simulink library "sm_excv_scene_lib"  (R2023a)
settings: Solver=VariableStepAuto  StartTime=0.0  StopTime=10.0  RelTol=1e-3
undefined symbols (not defined in the file): B1, B2, B3, B4, B5, B6, B7, B8, Excv, L1, L2, L3, L4, L5, L6, L7, L8, L9, Road, S1, S2, Scene, Scene_Data, SceneData, X, Y, Z
libraries: sm_lib x65, sm_tracked_vehicle_lib x47, $bdroot x45, nesl_utility x10
(part 1 of 3)
settings Model: Creator=smiller  LastModifiedBy=smiller

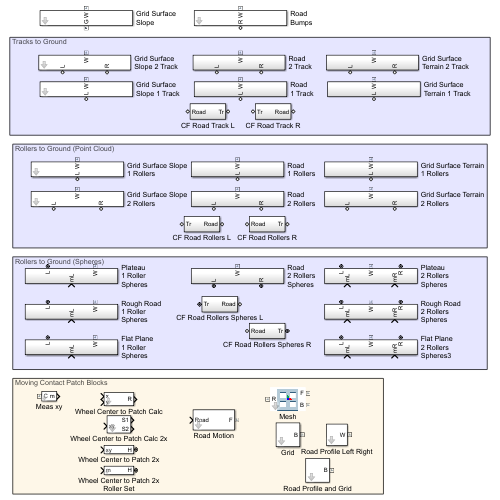
[thumbnail: Simulink's stored preview of the top-level diagram]
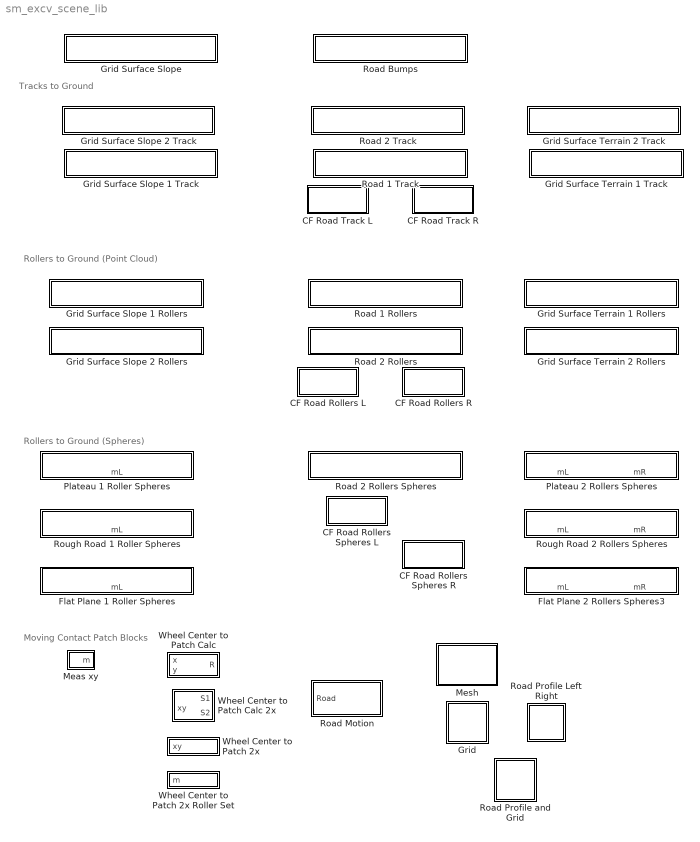
== system sm_excv_scene_lib ==
  note: Moving Contact Patch Blocks
  note: Rollers to Ground (Spheres)
  note: Tracks to Ground
  note: Rollers to Ground (Point Cloud)
  CF Road Rollers L : Subsystem
  CF Road Rollers R : Subsystem
  CF Road Rollers Spheres L : Subsystem
  CF Road Rollers Spheres R : Subsystem
  CF Road Track L : Subsystem
  CF Road Track R : Subsystem
  Flat Plane 1 Roller Spheres : Subsystem
  Flat Plane 2 Rollers Spheres3 : Subsystem
  Grid : Subsystem  VariantControl=Grid  mask(Grid){grid_x=SceneData.Grid.length, grid_y=SceneData.Grid.width, grid_z=SceneData.Grid.depth, grid_line_width=SceneData.Grid.linewidth, grid_num_sq_x=SceneData.Grid.numsquaresx, grid_num_sq_y=SceneData.Grid.numsquaresy, grid_clr=SceneData.Grid.linecolor, plane_clr=SceneData.Grid.planecolor, grid_opc=1}
      mask prompts: grid_x "Length (m) (Global x)"; grid_y "Width (m) (Global y)"; grid_z "Depth (m) (Global z)"; grid_line_width "Line width (m)"; grid_num_sq_x "Number of squares in x"; grid_num_sq_y "Number of squares in y"; grid_clr "Line Color [RGB]"; plane_clr "Plane Color [RGB]"; grid_opc "Opacity (0-1)"
      mask help: Creates a grid for use in animations.
      mask init:
      | % Derived parameters - for two perpendicular grids with num_sq-by-1 holes
      | % **Note, not num_sq_x by num_sq_y holes - better render speed with
      | % separate meshes for x and y.
      | 
      | hole_lx = (grid_x-(grid_line_width*(grid_num_sq_x+1)))/grid_num_sq_x;
      | hole_wx = (grid_y-(grid_line_width*(1+1)))/1;
      | 
      | hole_ly = (grid_y-(grid_line_width*(grid_num_sq_y+1)))/grid_num_sq_y;
      | hole_wy = (grid_x-(grid_line_width*(1+1)))/1;
  Grid Surface Slope : Subsystem  mask{road_len=Scene.Slope.road_len, road_wid=Scene.Slope.road_wid, slope_run=Scene.Slope.slope_run, slope_rise=Scene.Slope.slope_rise, slope_x0=Scene.Slope.slope_start, slope_xres=Scene.Slope.slope_xres, surface_clr=Scene.Slope.clr, surface_opc=Scene.Slope.opc}
      mask prompts: road_len "Road Length (m)"; road_wid "Road Width (m)"; slope_run "Slope Run(m)"; slope_rise "Slope Rise (m)"; slope_x0 "Slope Start (m)"; slope_xres "Slope Resolution (m)"; surface_clr "Color [R G B] (0-1)"; surface_opc "Opacity (0-1)"
      mask init:
      | gs_data = Grid_Surface_Data_Slope(road_len, road_wid, slope_run, slope_rise, slope_x0, slope_xres);
      mask TypeOptions surface_clr: Grid Surface/GraphicDiffuseColor
      mask TypeOptions surface_opc: Grid Surface/GraphicOpacity
  Grid Surface Slope 1 Track : Subsystem  mask{road_len=Scene.Slope.road_len, road_wid=Scene.Slope.road_wid, slope_rise=Scene.Slope.slope_rise, slope_run=Scene.Slope.slope_run, slope_x0=Scene.Slope.slope_start, slope_xres=Scene.Slope.slope_xres, surface_clr=Scene.Slope.clr, surface_opc=Scene.Slope.opc, K_Road=Scene.Contact.Terrain.K, B_Road=Scene.Contact.Terrain.B, TW_Road=Scene.Contact.Terrain.TW, F_dyn_Road=Scene.Contact.Terrain.mud, F_stat_Road=Scene.Contact.Terrain.mus, CV_Road=Scene.Contact.Terrain.CV}
      mask prompts: road_len "Road Length (m)"; road_wid "Road Width (m)"; slope_rise "Slope Rise (m)"; slope_run "Slope Run(m)"; slope_x0 "Slope Start (m)"; slope_xres "Slope Resolution (m)"; surface_clr "Color [R G B] (0-1)"; surface_opc "Opacity (0-1)"; K_Road "Normal Stiffness (N/m)"; B_Road "Normal Damping (N/(m/s))"; TW_Road "Normal Transition Width (m)"; F_dyn_Road "Coefficient of Dynamic Friction"; F_stat_Road "Coefficient of Static Friction"; CV_Road "Critical Velocity (m/s)"
      mask TypeOptions road_len:
      | Grid Surface
      | Slope/road_len
      mask TypeOptions road_wid:
      | Grid Surface
      | Slope/road_wid
      mask TypeOptions slope_rise:
      | Grid Surface
      | Slope/slope_rise
      mask TypeOptions slope_run:
      | Grid Surface
      | Slope/slope_run
      mask TypeOptions slope_x0:
      | Grid Surface
      | Slope/slope_x0
      mask TypeOptions slope_xres:
      | Grid Surface
      | Slope/slope_xres
      mask TypeOptions surface_clr:
      | Grid Surface
      | Slope/surface_clr
      mask TypeOptions surface_opc:
      | Grid Surface
      | Slope/surface_opc
      mask TypeOptions K_Road: CF Track Terrain L/K_Road
      mask TypeOptions B_Road: CF Track Terrain L/B_Road
      mask TypeOptions TW_Road: CF Track Terrain L/TW_Road
      mask TypeOptions F_dyn_Road: CF Track Terrain L/F_dyn_Road
      mask TypeOptions F_stat_Road: CF Track Terrain L/F_stat_Road
      mask TypeOptions CV_Road: CF Track Terrain L/CV_Road
      mask DialogControl cont_slope Prompt: Slope
      mask DialogControl cont_contact Prompt: Contact
  Grid Surface Slope 2 Track : Subsystem  mask{road_len=Scene.Slope.road_len, road_wid=Scene.Slope.road_wid, slope_rise=Scene.Slope.slope_rise, slope_run=Scene.Slope.slope_run, slope_x0=Scene.Slope.slope_start, slope_xres=Scene.Slope.slope_xres, surface_clr=Scene.Slope.clr, surface_opc=Scene.Slope.opc, TW_Road=Scene.Contact.Terrain.TW, B_Road=Scene.Contact.Terrain.B, K_Road=Scene.Contact.Terrain.K, F_dyn_Road=Scene.Contact.Terrain.mud, F_stat_Road=Scene.Contact.Terrain.mus, CV_Road=Scene.Contact.Terrain.CV}
      mask prompts: road_len "Road Length (m)"; road_wid "Road Width (m)"; slope_rise "Slope Rise (m)"; slope_run "Slope Run(m)"; slope_x0 "Slope Start (m)"; slope_xres "Slope Resolution (m)"; surface_clr "Color [R G B] (0-1)"; surface_opc "Opacity (0-1)"; TW_Road "Normal Transition Width (m)"; B_Road "Normal Damping (N/(m/s))"; K_Road "Normal Stiffness (N/m)"; F_dyn_Road "Coefficient of Dynamic Friction"; F_stat_Road "Coefficient of Static Friction"; CV_Road "Critical Velocity (m/s)"
      mask TypeOptions road_len:
      | Grid Surface
      | Slope/road_len
      mask TypeOptions road_wid:
      | Grid Surface
      | Slope/road_wid
      mask TypeOptions slope_rise:
      | Grid Surface
      | Slope/slope_rise
      mask TypeOptions slope_run:
      | Grid Surface
      | Slope/slope_run
      mask TypeOptions slope_x0:
      | Grid Surface
      | Slope/slope_x0
      mask TypeOptions slope_xres:
      | Grid Surface
      | Slope/slope_xres
      mask TypeOptions surface_clr:
      | Grid Surface
      | Slope/surface_clr
      mask TypeOptions surface_opc:
      | Grid Surface
      | Slope/surface_opc
      mask TypeOptions TW_Road: CF Track Terrain L/TW_Road | CF Track Terrain R/TW_Road
      mask TypeOptions B_Road: CF Track Terrain L/B_Road | CF Track Terrain R/B_Road
      mask TypeOptions K_Road: CF Track Terrain L/K_Road | CF Track Terrain R/K_Road
      mask TypeOptions F_dyn_Road: CF Track Terrain L/F_dyn_Road | CF Track Terrain R/F_dyn_Road
      mask TypeOptions F_stat_Road: CF Track Terrain L/F_stat_Road | CF Track Terrain R/F_stat_Road
      mask TypeOptions CV_Road: CF Track Terrain L/CV_Road | CF Track Terrain R/CV_Road
      mask DialogControl cont_slope Prompt: Slope
      mask DialogControl cont_contact Prompt: Contact
  Grid Surface Terrain 1 Track : Subsystem
  Grid Surface Terrain 2 Track : Subsystem
  Grid Surface Slope 1 Rollers : Subsystem  mask{road_len=Scene.Slope.road_len, road_wid=Scene.Slope.road_wid, slope_rise=Scene.Slope.slope_rise, slope_run=Scene.Slope.slope_run, slope_x0=Scene.Slope.slope_start, slope_xres=Scene.Slope.slope_xres, surface_clr=Scene.Slope.clr, surface_opc=Scene.Slope.opc, K_Road=Scene.Contact.Terrain.K, B_Road=Scene.Contact.Terrain.B, TW_Road=Scene.Contact.Terrain.TW, F_dyn_Road=Scene.Contact.Terrain.mud, F_stat_Road=Scene.Contact.Terrain.mus, CV_Road=Scene.Contact.Terrain.CV}
      mask prompts: road_len "Road Length (m)"; road_wid "Road Width (m)"; slope_rise "Slope Rise (m)"; slope_run "Slope Run(m)"; slope_x0 "Slope Start (m)"; slope_xres "Slope Resolution (m)"; surface_clr "Color [R G B] (0-1)"; surface_opc "Opacity (0-1)"; K_Road "Normal Stiffness (N/m)"; B_Road "Normal Damping (N/(m/s))"; TW_Road "Normal Transition Width (m)"; F_dyn_Road "Coefficient of Dynamic Friction"; F_stat_Road "Coefficient of Static Friction"; CV_Road "Critical Velocity (m/s)"
      mask TypeOptions road_len:
      | Grid Surface
      | Slope/road_len
      mask TypeOptions road_wid:
      | Grid Surface
      | Slope/road_wid
      mask TypeOptions slope_rise:
      | Grid Surface
      | Slope/slope_rise
      mask TypeOptions slope_run:
      | Grid Surface
      | Slope/slope_run
      mask TypeOptions slope_x0:
      | Grid Surface
      | Slope/slope_x0
      mask TypeOptions slope_xres:
      | Grid Surface
      | Slope/slope_xres
      mask TypeOptions surface_clr:
      | Grid Surface
      | Slope/surface_clr
      mask TypeOptions surface_opc:
      | Grid Surface
      | Slope/surface_opc
      mask TypeOptions K_Road: CF Track Terrain L/K_Road
      mask TypeOptions B_Road: CF Track Terrain L/B_Road
      mask TypeOptions TW_Road: CF Track Terrain L/TW_Road
      mask TypeOptions F_dyn_Road: CF Track Terrain L/F_dyn_Road
      mask TypeOptions F_stat_Road: CF Track Terrain L/F_stat_Road
      mask TypeOptions CV_Road: CF Track Terrain L/CV_Road
      mask DialogControl cont_slope Prompt: Slope
      mask DialogControl cont_contact Prompt: Contact
  Grid Surface Slope 2 Rollers : Subsystem  mask{road_len=Scene.Slope.road_len, road_wid=Scene.Slope.road_wid, slope_rise=Scene.Slope.slope_rise, slope_run=Scene.Slope.slope_run, slope_x0=Scene.Slope.slope_start, slope_xres=Scene.Slope.slope_xres, surface_clr=Scene.Slope.clr, surface_opc=Scene.Slope.opc, K_Road=Scene.Contact.Terrain.K, B_Road=Scene.Contact.Terrain.B, TW_Road=Scene.Contact.Terrain.TW, F_dyn_Road=Scene.Contact.Terrain.mud, F_stat_Road=Scene.Contact.Terrain.mus, CV_Road=Scene.Contact.Terrain.CV}
      mask prompts: road_len "Road Length (m)"; road_wid "Road Width (m)"; slope_rise "Slope Rise (m)"; slope_run "Slope Run(m)"; slope_x0 "Slope Start (m)"; slope_xres "Slope Resolution (m)"; surface_clr "Color [R G B] (0-1)"; surface_opc "Opacity (0-1)"; K_Road "Normal Stiffness (N/m)"; B_Road "Normal Damping (N/(m/s))"; TW_Road "Normal Transition Width (m)"; F_dyn_Road "Coefficient of Dynamic Friction"; F_stat_Road "Coefficient of Static Friction"; CV_Road "Critical Velocity (m/s)"
      mask TypeOptions road_len:
      | Grid Surface
      | Slope/road_len
      mask TypeOptions road_wid:
      | Grid Surface
      | Slope/road_wid
      mask TypeOptions slope_rise:
      | Grid Surface
      | Slope/slope_rise
      mask TypeOptions slope_run:
      | Grid Surface
      | Slope/slope_run
      mask TypeOptions slope_x0:
      | Grid Surface
      | Slope/slope_x0
      mask TypeOptions slope_xres:
      | Grid Surface
      | Slope/slope_xres
      mask TypeOptions surface_clr:
      | Grid Surface
      | Slope/surface_clr
      mask TypeOptions surface_opc:
      | Grid Surface
      | Slope/surface_opc
      mask TypeOptions K_Road: CF Track Terrain L/K_Road
      mask TypeOptions B_Road: CF Track Terrain L/B_Road
      mask TypeOptions TW_Road: CF Track Terrain L/TW_Road
      mask TypeOptions F_dyn_Road: CF Track Terrain L/F_dyn_Road
      mask TypeOptions F_stat_Road: CF Track Terrain L/F_stat_Road
      mask TypeOptions CV_Road: CF Track Terrain L/CV_Road
      mask DialogControl cont_slope Prompt: Slope
      mask DialogControl cont_contact Prompt: Contact
  Grid Surface Terrain 1 Rollers : Subsystem
  Grid Surface Terrain 2 Rollers : Subsystem
  Meas xy : Subsystem  mask(Measure Cartesian Location of two frames){whl_offset=Excv.Shoe.w}
      mask prompts: whl_offset "Frame Offset"
      mask help: Measure position of two frames. Frames are separated by a distance along their common z-axis.
  Mesh : Subsystem  mask(Rectangular Mesh){mesh_lenx=0.6, mesh_leny=0.4, mesh_hx=0.18, mesh_hy=0.18, mesh_numhx=3, mesh_numhy=2, mesh_thickness=0.02, mesh_rho=7000, mesh_color=[0 0.4 0.6], mesh_opc=1}
      mask prompts: mesh_thickness "Thickness (m)"; mesh_rho "Density (kg/m^3)"; mesh_color "Color [RGB]"; mesh_opc "Opacity (0-1)"
      mask help: Rectangular mesh. Define outer dimensions, dimensions of holes, and thickness. R port is at the CG. Thickness defines the distance of the F frame from the B frame along the z-axis.
      mask init:
      | mesh_xsec = sm_extr_data_mesh(mesh_lenx, mesh_leny, mesh_numhx, mesh_numhy, mesh_hx, mesh_hy);
      mask DialogControl Control12 Prompt: Plot Profile
      mask DialogControl Control12 Callback:
      | v = get_param(gcb,'MaskWSVariables');
      | getMaskValue = containers.Map({v.Name}',{v.Value}');
      | evalin('base',...
      |     sprintf('Extr_Data_Mesh(%s,%s,%s,%s,%s,%s,''%s'');',...
      |     num2str(getMaskValue('mesh_lenx')),...
      |     num2str(getMaskValue('mesh_leny')),...
      |     num2str(getMaskValue('mesh_numhx')),...
      |     num2str(getMaskValue('mesh_numhy')),...
      |     num2str(getMaskValue('mesh_hx')),...
      |     num2str(getMaskValue('mesh_hy')),'plot'));
      mask DialogControl Control7 Prompt: X
      mask DialogControl Control8 Prompt: Y
      mask DialogControl Control9 Prompt: Mesh Length (m)
      mask DialogControl Control11 Prompt: Hole Length (m)
      mask DialogControl Control10 Prompt: Number of Holes
      mask Display: image('sm_parts_mesh_image.png');
  Plateau 1 Roller Spheres : Subsystem
  Plateau 2 Rollers Spheres : Subsystem
  Road 1 Rollers : Subsystem
  Road 1 Track : Subsystem
  Road 2 Rollers : Subsystem
  Road 2 Rollers Spheres : Subsystem
  Road 2 Track : Subsystem
  Road Bumps : Subsystem  mask{road_x=Scene.Road.len, road_y=Scene.Road.wid, road_z=Scene.Road.hgt, bump_x=Scene.Road.Bump.len, bump_y=Scene.Road.Bump.wid, bump_z=Scene.Road.Bump.hgt, bloc_y=Scene.Road.Bump.offsety, bloc_z=Scene.Road.Bump.offsetz, bump_x0=Scene.Road.Bump.startx, bloc_dx=Scene.Road.Bump.deltax}
      mask prompts: road_x "Length (m)"; road_y "Width (m)"; road_z "Thickness (m)"; bump_x "Length (m)"; bump_y "Width (m)"; bump_z "Height (m)"; bloc_y "Offset y (m)"; bloc_z "Offset z (m)"; bump_x0 "Start x (m)"; bloc_dx "Spacing x (m)"
      mask DialogControl cont_road Prompt: Road
      mask DialogControl cont_bump_dim Prompt: Bump
      mask DialogControl cont_bump_offset Prompt: Bump Offset
  Road Motion : Subsystem  mask(Position Infinite Plane){}
      mask help: Positions and orients Infinite Plane based on input signal. Abstract method of modeling objects contacting uneven terrain.
  Road Profile Left Right : Subsystem  mask(Left and Right Paths for Wheels.){RDF_Polyline=Scene_Data.Plateau}
      mask prompts: RDF_Polyline "RDF Polyline (structure)"
      mask help: Creates left and right straightline paths for wheels as an extrusion. Look under mask to see the format of the structure required.
  Road Profile and Grid : Subsystem  VariantControl=Plateau  mask(Display Wheel Paths and Grid){RDF_Polyline=Scene.Plateau, grid_z_offset=-0.2, grid_x=Scene.Grid.length, grid_y=Scene.Grid.width, grid_z=Scene.Grid.depth, grid_line_width=Scene.Grid.linewidth, grid_num_sq_x=Scene.Grid.numsquaresx, grid_num_sq_y=Scene.Grid.numsquaresy, plane_clr=Scene.Grid.planecolor, grid_clr=Scene.Grid.linecolor, grid_opc=1}
      mask prompts: RDF_Polyline "Road Data (structure)"; grid_z_offset "Offset Grid in z (m)"; grid_x "Length (m) (Global x)"; grid_y "Width (m) (Global y)"; grid_z "Depth (m) (Global z)"; grid_line_width "Line width (m)"; grid_num_sq_x "Number of squares in x"; grid_num_sq_y "Number of squares in y"; plane_clr "Plane Color [RGB]"; grid_clr "Line Color [RGB]"; grid_opc "Opacity (0-1)"
      mask help: Display wheel paths and grid.
      mask init: same as sm_excv_scene_lib/Grid
      mask TypeOptions RDF_Polyline: Plateau/RDF_Polyline
      mask TypeOptions grid_x: Grid/grid_x
      mask TypeOptions grid_y: Grid/grid_y
      mask TypeOptions grid_z: Grid/grid_z
      mask TypeOptions grid_line_width: Grid/grid_line_width
      mask TypeOptions grid_num_sq_x: Grid/grid_num_sq_x
      mask TypeOptions grid_num_sq_y: Grid/grid_num_sq_y
      mask TypeOptions plane_clr: Grid/plane_clr
      mask TypeOptions grid_clr: Grid/grid_clr
      mask TypeOptions grid_opc: Grid/grid_opc
      mask DialogControl cont_grid Prompt: Grid Parameters
  Rough Road 1 Roller Spheres : Subsystem
  Rough Road 2 Rollers Spheres : Subsystem
  Wheel Center to Patch 2x : Subsystem  mask(Wheel Center to Patch Height and Pitch, Infinite Planes){road_pz_x=Scene.Plateau.Road.pzLUT.px, road_pz_z=Scene.Plateau.Road.pzLUT.pz(:,1), road_qy_x=Scene.Plateau.Road.qyLUT.px, road_qy_qy=Scene.Plateau.Road.qyLUT.qy(:,1), tfilter=0.01, patch_clr=[0.5 0.5 0.5], patch_opc=0.25, patch_x=1, patch_y=1, NormalStiffness=Scene.Contact.Terrain.K, NormalDamping=Scene.Contact.Terrain.B, NormalTransitionRegionWidth=Scene.Contact.Terrain.TW, CoefficientOfDynamicFriction=Scene.Contact.Terrain.mud, CoefficientOfStaticFriction=Scene.Contact.Terrain.mus, FrictionalCriticalVelocity=Scene.Contact.Terrain.CV}
      mask prompts: road_pz_x "Road Distances (m)"; road_pz_z "Road Heights (m)"; road_qy_x "Road Distances(m)"; road_qy_qy "Road Pitch (m)"; tfilter "Filter Constant (seconds)"; patch_clr "Color [R G B] (0-1)"; patch_opc "Opacity (0-1)"; patch_x "Patch Length x (m)"; patch_y "Patch Length y (m)"; NormalStiffness "Normal Stiffness (N/m)"; NormalDamping "Normal Damping (N/(m/s))"; NormalTransitionRegionWidth "Normal Transition Width (m)"; CoefficientOfDynamicFriction "Coefficient of Dynamic Friction"; CoefficientOfStaticFriction "Coefficient of Static Friction"; FrictionalCriticalVelocity "Critical Velocity (m/s)"
      mask help: Find contact patch height and pitch using a lookup table, where the inputs are the x-y location of two frames. The output is a Simscape Bus with the geometry ports for Infinite Planes positioned and pitched for the two input frame locations.
      mask TypeOptions road_pz_x:
      | Wheel Center
      | to Patch/road_pz_x
      mask TypeOptions road_pz_z:
      | Wheel Center
      | to Patch/road_pz_z
      mask TypeOptions road_qy_x:
      | Wheel Center
      | to Patch/road_qy_x
      mask TypeOptions road_qy_qy:
      | Wheel Center
      | to Patch/road_qy_qy
      mask TypeOptions tfilter:
      | Wheel Center
      | to Patch/tfilter
      mask TypeOptions patch_clr: Infinite Plane1/GraphicDiffuseColor | Infinite Plane2/GraphicDiffuseColor
      mask TypeOptions patch_opc: Infinite Plane1/GraphicOpacity | Infinite Plane2/GraphicOpacity
      mask TypeOptions patch_x: Infinite Plane1/GraphicPlaneWidth | Infinite Plane2/GraphicPlaneWidth
      mask TypeOptions patch_y: Infinite Plane1/GraphicPlaneHeight | Infinite Plane2/GraphicPlaneHeight
      mask TypeOptions NormalStiffness: CF Track Terrain1/NormalStiffness | CF Track Terrain2/NormalStiffness
      mask TypeOptions NormalDamping: CF Track Terrain1/NormalDamping | CF Track Terrain2/NormalDamping
      mask TypeOptions NormalTransitionRegionWidth: CF Track Terrain1/NormalTransitionRegionWidth | CF Track Terrain2/NormalTransitionRegionWidth
      mask TypeOptions CoefficientOfDynamicFriction: CF Track Terrain1/CoefficientOfDynamicFriction | CF Track Terrain2/CoefficientOfDynamicFriction
      mask TypeOptions CoefficientOfStaticFriction: CF Track Terrain1/CoefficientOfStaticFriction | CF Track Terrain2/CoefficientOfStaticFriction
      mask TypeOptions FrictionalCriticalVelocity: CF Track Terrain1/FrictionalCriticalVelocity | CF Track Terrain2/FrictionalCriticalVelocity
      mask DialogControl cont_surface Prompt: Surface
      mask DialogControl cont_patchvis Prompt: Patch Visual
      mask DialogControl cont_contact Prompt: Contact
  Wheel Center to Patch 2x Roller Set : Subsystem  mask(Wheel Center to Patch Height and Pitch, All Rollers){road_pz_x=Scene.Plateau.Road.pzLUT.px, road_pz_z=Scene.Plateau.Road.pzLUT.pz(:,1), road_qy_x=Scene.Plateau.Road.qyLUT.px, road_qy_qy=Scene.Plateau.Road.qyLUT.qy(:,1), tfilter=0.01, NormalStiffness=Scene.Contact.Terrain.K, NormalDamping=Scene.Contact.Terrain.B, NormalTransitionRegionWidth=Scene.Contact.Terrain.TW, CoefficientOfDynamicFriction=Scene.Contact.Terrain.mud, CoefficientOfStaticFriction=Scene.Contact.Terrain.mus, FrictionalCriticalVelocity=Scene.Contact.Terrain.CV, patch_x=1, patch_y=1, patch_clr=[0.5 0.5 0.5], patch_opc=0.25}
      mask prompts: road_pz_x "Road Distances (m)"; road_pz_z "Road Heights (m)"; road_qy_x "Road Distances(m)"; road_qy_qy "Road Pitch (m)"; tfilter "Filter Constant (seconds)"; NormalStiffness "Normal Stiffness (N/m)"; NormalDamping "Normal Damping (N/(m/s))"; NormalTransitionRegionWidth "Normal Transition Width (m)"; CoefficientOfDynamicFriction "Coefficient of Dynamic Friction"; CoefficientOfStaticFriction "Coefficient of Static Friction"; FrictionalCriticalVelocity "Critical Velocity (m/s)"; patch_x "Patch Length x (m)"; patch_y "Patch Length y (m)"; patch_clr "Color [R G B] (0-1)"; patch_opc "Opacity (0-1)"
      mask help: Find contact patch height and pitch using a lookup table, where the inputs are the x-y location of two frames. The output is a Simscape Bus with the geometry ports for Infinite Planes positioned and pitched for all input frame locations.
      mask TypeOptions road_pz_x: Wheel Center to Patch Contact 1/road_pz_x | Wheel Center to Patch Contact 2/road_pz_x | Wheel Center to Patch Contact 3/road_pz_x | Wheel Center to Patch Contact 4/road_pz_x | Wheel Center to Patch Contact 5/road_pz_x | Wheel Center to Patch Contact 6/road_pz_x | Wheel Center to Patch Contact 7/road_pz_x | Wheel Center to Patch Contact 8/road_pz_x | Wheel Center to Patch Contact 9/road_pz_x
      mask TypeOptions road_pz_z: Wheel Center to Patch Contact 1/road_pz_z | Wheel Center to Patch Contact 2/road_pz_z | Wheel Center to Patch Contact 3/road_pz_z | Wheel Center to Patch Contact 4/road_pz_z | Wheel Center to Patch Contact 5/road_pz_z | Wheel Center to Patch Contact 6/road_pz_z | Wheel Center to Patch Contact 7/road_pz_z | Wheel Center to Patch Contact 8/road_pz_z | Wheel Center to Patch Contact 9/road_pz_z
      mask TypeOptions road_qy_x: Wheel Center to Patch Contact 1/road_qy_x | Wheel Center to Patch Contact 2/road_qy_x | Wheel Center to Patch Contact 3/road_qy_x | Wheel Center to Patch Contact 4/road_qy_x | Wheel Center to Patch Contact 5/road_qy_x | Wheel Center to Patch Contact 6/road_qy_x | Wheel Center to Patch Contact 7/road_qy_x | Wheel Center to Patch Contact 8/road_qy_x | Wheel Center to Patch Contact 9/road_qy_x
      mask TypeOptions road_qy_qy: Wheel Center to Patch Contact 1/road_qy_qy | Wheel Center to Patch Contact 2/road_qy_qy | Wheel Center to Patch Contact 3/road_qy_qy | Wheel Center to Patch Contact 4/road_qy_qy | Wheel Center to Patch Contact 5/road_qy_qy | Wheel Center to Patch Contact 6/road_qy_qy | Wheel Center to Patch Contact 7/road_qy_qy | Wheel Center to Patch Contact 8/road_qy_qy | Wheel Center to Patch Contact 9/road_qy_qy
      mask TypeOptions tfilter: Wheel Center to Patch Contact 1/tfilter | Wheel Center to Patch Contact 2/tfilter | Wheel Center to Patch Contact 3/tfilter | Wheel Center to Patch Contact 4/tfilter | Wheel Center to Patch Contact 5/tfilter | Wheel Center to Patch Contact 6/tfilter | Wheel Center to Patch Contact 7/tfilter | Wheel Center to Patch Contact 8/tfilter | Wheel Center to Patch Contact 9/tfilter
      mask TypeOptions NormalStiffness: Wheel Center to Patch Contact 1/NormalStiffness | Wheel Center to Patch Contact 2/NormalStiffness | Wheel Center to Patch Contact 3/NormalStiffness | Wheel Center to Patch Contact 4/NormalStiffness | Wheel Center to Patch Contact 5/NormalStiffness | Wheel Center to Patch Contact 6/NormalStiffness | Wheel Center to Patch Contact 7/NormalStiffness | Wheel Center to Patch Contact 8/NormalStiffness | Wheel Center to Patch Contact 9/NormalStiffness
      mask TypeOptions NormalDamping: Wheel Center to Patch Contact 1/NormalDamping | Wheel Center to Patch Contact 2/NormalDamping | Wheel Center to Patch Contact 3/NormalDamping | Wheel Center to Patch Contact 4/NormalDamping | Wheel Center to Patch Contact 5/NormalDamping | Wheel Center to Patch Contact 6/NormalDamping | Wheel Center to Patch Contact 7/NormalDamping | Wheel Center to Patch Contact 8/NormalDamping | Wheel Center to Patch Contact 9/NormalDamping
      mask TypeOptions NormalTransitionRegionWidth: Wheel Center to Patch Contact 1/NormalTransitionRegionWidth | Wheel Center to Patch Contact 2/NormalTransitionRegionWidth | Wheel Center to Patch Contact 3/NormalTransitionRegionWidth | Wheel Center to Patch Contact 4/NormalTransitionRegionWidth | Wheel Center to Patch Contact 5/NormalTransitionRegionWidth | Wheel Center to Patch Contact 6/NormalTransitionRegionWidth | Wheel Center to Patch Contact 7/NormalTransitionRegionWidth | Wheel Center to Patch Contact 8/NormalTransitionRegionWidth | Wheel Center to Patch Contact 9/NormalTransitionRegionWidth
      mask TypeOptions CoefficientOfDynamicFriction: Wheel Center to Patch Contact 1/CoefficientOfDynamicFriction | Wheel Center to Patch Contact 2/CoefficientOfDynamicFriction | Wheel Center to Patch Contact 3/CoefficientOfDynamicFriction | Wheel Center to Patch Contact 4/CoefficientOfDynamicFriction | Wheel Center to Patch Contact 5/CoefficientOfDynamicFriction | Wheel Center to Patch Contact 6/CoefficientOfDynamicFriction | Wheel Center to Patch Contact 7/CoefficientOfDynamicFriction | Wheel Center to Patch Contact 8/CoefficientOfDynamicFriction | Wheel Center to Patch Contact 9/CoefficientOfDynamicFriction
      mask TypeOptions CoefficientOfStaticFriction: Wheel Center to Patch Contact 1/CoefficientOfStaticFriction | Wheel Center to Patch Contact 2/CoefficientOfStaticFriction | Wheel Center to Patch Contact 3/CoefficientOfStaticFriction | Wheel Center to Patch Contact 4/CoefficientOfStaticFriction | Wheel Center to Patch Contact 5/CoefficientOfStaticFriction | Wheel Center to Patch Contact 6/CoefficientOfStaticFriction | Wheel Center to Patch Contact 7/CoefficientOfStaticFriction | Wheel Center to Patch Contact 8/CoefficientOfStaticFriction | Wheel Center to Patch Contact 9/CoefficientOfStaticFriction
      mask TypeOptions FrictionalCriticalVelocity: Wheel Center to Patch Contact 1/FrictionalCriticalVelocity | Wheel Center to Patch Contact 2/FrictionalCriticalVelocity | Wheel Center to Patch Contact 3/FrictionalCriticalVelocity | Wheel Center to Patch Contact 4/FrictionalCriticalVelocity | Wheel Center to Patch Contact 5/FrictionalCriticalVelocity | Wheel Center to Patch Contact 6/FrictionalCriticalVelocity | Wheel Center to Patch Contact 7/FrictionalCriticalVelocity | Wheel Center to Patch Contact 8/FrictionalCriticalVelocity | Wheel Center to Patch Contact 9/FrictionalCriticalVelocity
      mask TypeOptions patch_x: Wheel Center to Patch Contact 1/patch_x | Wheel Center to Patch Contact 2/patch_x | Wheel Center to Patch Contact 3/patch_x | Wheel Center to Patch Contact 4/patch_x | Wheel Center to Patch Contact 5/patch_x | Wheel Center to Patch Contact 6/patch_x | Wheel Center to Patch Contact 7/patch_x | Wheel Center to Patch Contact 8/patch_x | Wheel Center to Patch Contact 9/patch_x
      mask TypeOptions patch_y: Wheel Center to Patch Contact 1/patch_y | Wheel Center to Patch Contact 2/patch_y | Wheel Center to Patch Contact 3/patch_y | Wheel Center to Patch Contact 4/patch_y | Wheel Center to Patch Contact 5/patch_y | Wheel Center to Patch Contact 6/patch_y | Wheel Center to Patch Contact 7/patch_y | Wheel Center to Patch Contact 8/patch_y | Wheel Center to Patch Contact 9/patch_y
      mask TypeOptions patch_clr: Wheel Center to Patch Contact 1/patch_clr | Wheel Center to Patch Contact 2/patch_clr | Wheel Center to Patch Contact 3/patch_clr | Wheel Center to Patch Contact 4/patch_clr | Wheel Center to Patch Contact 5/patch_clr | Wheel Center to Patch Contact 6/patch_clr | Wheel Center to Patch Contact 7/patch_clr | Wheel Center to Patch Contact 8/patch_clr | Wheel Center to Patch Contact 9/patch_clr
      mask TypeOptions patch_opc: Wheel Center to Patch Contact 1/patch_opc | Wheel Center to Patch Contact 2/patch_opc | Wheel Center to Patch Contact 3/patch_opc | Wheel Center to Patch Contact 4/patch_opc | Wheel Center to Patch Contact 5/patch_opc | Wheel Center to Patch Contact 6/patch_opc | Wheel Center to Patch Contact 7/patch_opc | Wheel Center to Patch Contact 8/patch_opc | Wheel Center to Patch Contact 9/patch_opc
      mask DialogControl cont_surface Prompt: Surface
      mask DialogControl cont_surfHeight Prompt: Height
      mask DialogControl cont_surfPitch Prompt: Pitch
      mask DialogControl cont_contact Prompt: Contact
      mask DialogControl cont_patchvis Prompt: Patch Visual
  Wheel Center to Patch Calc : Subsystem  mask(Wheel Center to Patch Height and Pitch){road_pz_x=Scene.Plateau.Road.pzLUT.px, road_pz_z=Scene.Plateau.Road.pzLUT.pz(:,1), road_qy_x=Scene.Plateau.Road.qyLUT.px, road_qy_qy=Scene.Plateau.Road.qyLUT.qy(:,1)}
      mask prompts: road_pz_x "Road Distances (m)"; road_pz_z "Road Heights (m)"; road_qy_x "Road Distances(m)"; road_qy_qy "Road Pitch (m)"
      mask help: Find contact patch height and pitch using a lookup table, where the inputs are the x-y location of the frame.
      mask DialogControl cont_roadpz Prompt: Road Height
      mask DialogControl cont_roadqy Prompt: Road Pitch
  Wheel Center to Patch Calc 2x : Subsystem  mask(Wheel Center to Patch Height and Pitch, Two Frames){road_pz_x=Scene.Plateau.Road.pzLUT.px, road_pz_z=Scene.Plateau.Road.pzLUT.pz(:,1), road_qy_x=Scene.Plateau.Road.qyLUT.px, road_qy_qy=Scene.Plateau.Road.qyLUT.qy(:,1), tfilter=0.01}
      mask prompts: road_pz_x "Road Distances (m)"; road_pz_z "Road Heights (m)"; road_qy_x "Road Distances(m)"; road_qy_qy "Road Pitch (m)"; tfilter "Filter Constant (seconds)"
      mask help: Find contact patch height and pitch using a lookup table, where the inputs are the x-y location of two frames.
      mask TypeOptions road_pz_x: Wheel Center to Patch1/road_pz_x | Wheel Center to Patch2/road_pz_x
      mask TypeOptions road_pz_z: Wheel Center to Patch1/road_pz_z | Wheel Center to Patch2/road_pz_z
      mask TypeOptions road_qy_x: Wheel Center to Patch1/road_qy_x | Wheel Center to Patch2/road_qy_x
      mask TypeOptions road_qy_qy: Wheel Center to Patch1/road_qy_qy | Wheel Center to Patch2/road_qy_qy

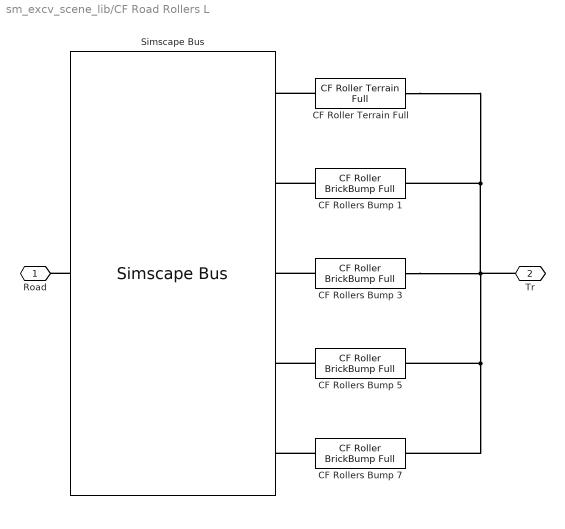
== system sm_excv_scene_lib/CF Road Rollers L ==
  CF Roller Terrain Full : sm_tracked_vehicle_lib/CF Roller Terrain Full  K_Road=Scene.Contact.Terrain.K  B_Road=Scene.Contact.Terrain.B  TW_Road=Scene.Contact.Terrain.TW  F_dyn_Road=Scene.Contact.Terrain.mud  F_stat_Road=Scene.Contact.Terrain.mus  CV_Road=Scene.Contact.Terrain.CV
  "CF Rollers Bump 1 " : sm_tracked_vehicle_lib/CF Roller BrickBump Full  K_BrickBump=Scene.Contact.BrickBump.K  B_BrickBump=Scene.Contact.BrickBump.B  TW_BrickBump=Scene.Contact.BrickBump.TW
  CF Rollers Bump 3 : sm_tracked_vehicle_lib/CF Roller BrickBump Full  K_BrickBump=Scene.Contact.BrickBump.K  B_BrickBump=Scene.Contact.BrickBump.B  TW_BrickBump=Scene.Contact.BrickBump.TW
  CF Rollers Bump 5 : sm_tracked_vehicle_lib/CF Roller BrickBump Full  K_BrickBump=Scene.Contact.BrickBump.K  B_BrickBump=Scene.Contact.BrickBump.B  TW_BrickBump=Scene.Contact.BrickBump.TW
  CF Rollers Bump 7 : sm_tracked_vehicle_lib/CF Roller BrickBump Full  K_BrickBump=Scene.Contact.BrickBump.K  B_BrickBump=Scene.Contact.BrickBump.B  TW_BrickBump=Scene.Contact.BrickBump.TW
  Simscape Bus : SimscapeBus  HierarchyStrings=Road;B1;B3;B5;B7  ConnectionType=Bus: Road_CBO
  Road : PMIOPort  Side=Left
  Tr : PMIOPort  Port=2  Side=Right
  connections:
  CF Rollers Bump 3/LConn1 -- Simscape Bus/LConn3
  "CF Rollers Bump 1 "/LConn1 -- Simscape Bus/LConn2
  CF Roller Terrain Full/LConn1 -- Simscape Bus/LConn1
  Simscape Bus/RConn1 -- Road/RConn1
  CF Rollers Bump 5/LConn1 -- Simscape Bus/LConn4
  CF Rollers Bump 7/LConn1 -- Simscape Bus/LConn5
  Tr/RConn1 -- CF Rollers Bump 3/RConn1 -- CF Roller Terrain Full/RConn1 -- "CF Rollers Bump 1 "/RConn1 -- CF Rollers Bump 5/RConn1 -- CF Rollers Bump 7/RConn1

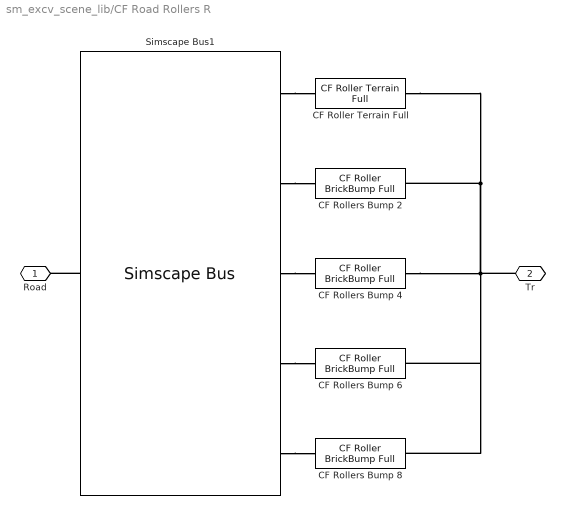
== system sm_excv_scene_lib/CF Road Rollers R ==
  CF Roller Terrain Full : sm_tracked_vehicle_lib/CF Roller Terrain Full  K_Road=Scene.Contact.Terrain.K  B_Road=Scene.Contact.Terrain.B  TW_Road=Scene.Contact.Terrain.TW  F_dyn_Road=Scene.Contact.Terrain.mud  F_stat_Road=Scene.Contact.Terrain.mus  CV_Road=Scene.Contact.Terrain.CV
  "CF Rollers Bump 2 " : sm_tracked_vehicle_lib/CF Roller BrickBump Full  K_BrickBump=Scene.Contact.BrickBump.K  B_BrickBump=Scene.Contact.BrickBump.B  TW_BrickBump=Scene.Contact.BrickBump.TW
  CF Rollers Bump 4 : sm_tracked_vehicle_lib/CF Roller BrickBump Full  K_BrickBump=Scene.Contact.BrickBump.K  B_BrickBump=Scene.Contact.BrickBump.B  TW_BrickBump=Scene.Contact.BrickBump.TW
  CF Rollers Bump 6 : sm_tracked_vehicle_lib/CF Roller BrickBump Full  K_BrickBump=Scene.Contact.BrickBump.K  B_BrickBump=Scene.Contact.BrickBump.B  TW_BrickBump=Scene.Contact.BrickBump.TW
  CF Rollers Bump 8 : sm_tracked_vehicle_lib/CF Roller BrickBump Full  K_BrickBump=Scene.Contact.BrickBump.K  B_BrickBump=Scene.Contact.BrickBump.B  TW_BrickBump=Scene.Contact.BrickBump.TW
  Simscape Bus1 : SimscapeBus  HierarchyStrings=Road;B2;B4;B6;B8  ConnectionType=Bus: Road_CBO
  Road : PMIOPort  Side=Left
  Tr : PMIOPort  Port=2  Side=Right
  connections:
  CF Roller Terrain Full/RConn1 -- "CF Rollers Bump 2 "/RConn1 -- CF Rollers Bump 8/RConn1 -- CF Rollers Bump 6/RConn1 -- Tr/RConn1 -- CF Rollers Bump 4/RConn1
  Simscape Bus1/LConn5 -- CF Rollers Bump 8/LConn1
  Simscape Bus1/LConn4 -- CF Rollers Bump 6/LConn1
  Simscape Bus1/RConn1 -- Road/RConn1
  Simscape Bus1/LConn1 -- CF Roller Terrain Full/LConn1
  Simscape Bus1/LConn2 -- "CF Rollers Bump 2 "/LConn1
  Simscape Bus1/LConn3 -- CF Rollers Bump 4/LConn1

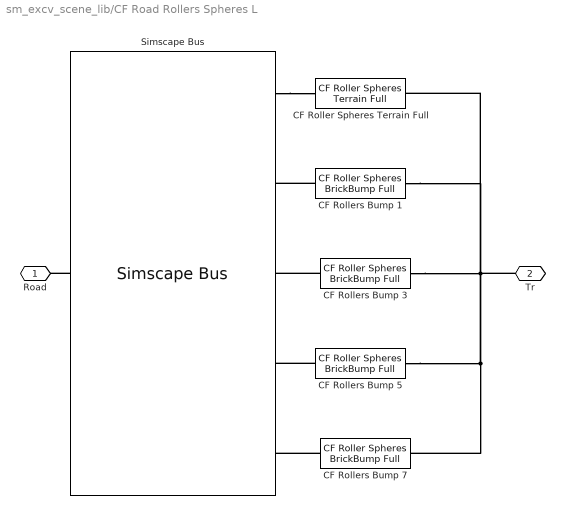
== system sm_excv_scene_lib/CF Road Rollers Spheres L ==
  CF Roller Spheres Terrain Full : sm_tracked_vehicle_lib/CF Roller Spheres Terrain Full  K_Road=Scene.Contact.Terrain.K  B_Road=Scene.Contact.Terrain.B  TW_Road=Scene.Contact.Terrain.TW  F_dyn_Road=Scene.Contact.Terrain.mud  F_stat_Road=Scene.Contact.Terrain.mus  CV_Road=Scene.Contact.Terrain.CV
  CF Rollers Bump {1,3,5,7} (4 alike) : sm_tracked_vehicle_lib/CF Roller Spheres BrickBump Full  K_BrickBump=Scene.Contact.BrickBump.K  B_BrickBump=Scene.Contact.BrickBump.B  TW_BrickBump=Scene.Contact.BrickBump.TW
  Simscape Bus : SimscapeBus  HierarchyStrings=Road;B1;B3;B5;B7  ConnectionType=Bus: Road_CBO
  Road : PMIOPort  Side=Left
  Tr : PMIOPort  Port=2  Side=Right
  connections:
  Tr/RConn1 -- CF Rollers Bump 3/RConn1 -- CF Roller Spheres Terrain Full/RConn1 -- CF Rollers Bump 1/RConn1 -- CF Rollers Bump 7/RConn1 -- CF Rollers Bump 5/RConn1
  CF Rollers Bump 7/LConn1 -- Simscape Bus/LConn5
  CF Rollers Bump 5/LConn1 -- Simscape Bus/LConn4
  Simscape Bus/RConn1 -- Road/RConn1
  Simscape Bus/LConn1 -- CF Roller Spheres Terrain Full/LConn1
  CF Rollers Bump 1/LConn1 -- Simscape Bus/LConn2
  CF Rollers Bump 3/LConn1 -- Simscape Bus/LConn3

== system sm_excv_scene_lib/CF Road Rollers Spheres R ==
  CF Roller Spheres Terrain Full : sm_tracked_vehicle_lib/CF Roller Spheres Terrain Full  K_Road=Scene.Contact.Terrain.K  B_Road=Scene.Contact.Terrain.B  TW_Road=Scene.Contact.Terrain.TW  F_dyn_Road=Scene.Contact.Terrain.mud  F_stat_Road=Scene.Contact.Terrain.mus  CV_Road=Scene.Contact.Terrain.CV
  CF Rollers Bump {1,3,5,7} (4 alike) : sm_tracked_vehicle_lib/CF Roller Spheres BrickBump Full  K_BrickBump=Scene.Contact.BrickBump.K  B_BrickBump=Scene.Contact.BrickBump.B  TW_BrickBump=Scene.Contact.BrickBump.TW
  Simscape Bus1 : SimscapeBus  HierarchyStrings=Road;B2;B4;B6;B8  ConnectionType=Bus: Road_CBO
  Road : PMIOPort  Side=Left
  Tr : PMIOPort  Port=2  Side=Right
  connections:
  Simscape Bus1/LConn3 -- CF Rollers Bump 3/LConn1
  Simscape Bus1/LConn2 -- CF Rollers Bump 1/LConn1
  CF Roller Spheres Terrain Full/LConn1 -- Simscape Bus1/LConn1
  Simscape Bus1/RConn1 -- Road/RConn1
  Simscape Bus1/LConn4 -- CF Rollers Bump 5/LConn1
  Simscape Bus1/LConn5 -- CF Rollers Bump 7/LConn1
  CF Rollers Bump 7/RConn1 -- CF Roller Spheres Terrain Full/RConn1 -- CF Rollers Bump 1/RConn1 -- CF Rollers Bump 3/RConn1 -- Tr/RConn1 -- CF Rollers Bump 5/RConn1

== system sm_excv_scene_lib/CF Road Track L ==
  CF Track Bump {1,3,5,7} (4 alike) : sm_tracked_vehicle_lib/CF Track BrickBump Full  K_BrickBump=Scene.Contact.BrickBump.K  B_BrickBump=Scene.Contact.BrickBump.B  TW_BrickBump=Scene.Contact.BrickBump.TW
      settings: LibrarySourceBlock=sm_chain_drive_lib/CF_BrickBump_Full
  CF Track Terrain : sm_tracked_vehicle_lib/CF Track Terrain Full  K_Road=Scene.Contact.Terrain.K  B_Road=Scene.Contact.Terrain.B  TW_Road=Scene.Contact.Terrain.TW  F_dyn_Road=Scene.Contact.Terrain.mud  F_stat_Road=Scene.Contact.Terrain.mus  CV_Road=Scene.Contact.Terrain.CV
      settings: LibrarySourceBlock=sm_chain_drive_lib/CF_Road_Full
  Simscape Bus : SimscapeBus  HierarchyStrings=Road;B1;B3;B5;B7  ConnectionType=Bus: Road_CBO
  Road : PMIOPort  Side=Left
  Tr : PMIOPort  Port=2  Side=Right
  connections:
  CF Track Terrain/RConn1 -- CF Track Bump 3/RConn1 -- CF Track Bump 5/RConn1 -- CF Track Bump 7/RConn1 -- Tr/RConn1 -- CF Track Bump 1/RConn1
  Simscape Bus/LConn5 -- CF Track Bump 7/LConn1
  Simscape Bus/LConn4 -- CF Track Bump 5/LConn1
  Simscape Bus/RConn1 -- Road/RConn1
  Simscape Bus/LConn1 -- CF Track Terrain/LConn1
  Simscape Bus/LConn2 -- CF Track Bump 1/LConn1
  Simscape Bus/LConn3 -- CF Track Bump 3/LConn1

== system sm_excv_scene_lib/CF Road Track R ==
  CF Track Bump {2,4,6,8} (4 alike) : sm_tracked_vehicle_lib/CF Track BrickBump Full  K_BrickBump=Scene.Contact.BrickBump.K  B_BrickBump=Scene.Contact.BrickBump.B  TW_BrickBump=Scene.Contact.BrickBump.TW
      settings: LibrarySourceBlock=sm_chain_drive_lib/CF_BrickBump_Full
  CF Track Terrain : sm_tracked_vehicle_lib/CF Track Terrain Full  K_Road=Scene.Contact.Terrain.K  B_Road=Scene.Contact.Terrain.B  TW_Road=Scene.Contact.Terrain.TW  F_dyn_Road=Scene.Contact.Terrain.mud  F_stat_Road=Scene.Contact.Terrain.mus  CV_Road=Scene.Contact.Terrain.CV
      settings: LibrarySourceBlock=sm_chain_drive_lib/CF_Road_Full
  Simscape Bus1 : SimscapeBus  HierarchyStrings=Road;B2;B4;B6;B8  ConnectionType=Bus: Road_CBO
  Road : PMIOPort  Side=Left
  Tr : PMIOPort  Port=2  Side=Right
  connections:
  Simscape Bus1/LConn3 -- CF Track Bump 4/LConn1
  Simscape Bus1/LConn2 -- CF Track Bump 2/LConn1
  Simscape Bus1/LConn1 -- CF Track Terrain/LConn1
  Simscape Bus1/RConn1 -- Road/RConn1
  Simscape Bus1/LConn4 -- CF Track Bump 6/LConn1
  Simscape Bus1/LConn5 -- CF Track Bump 8/LConn1
  Tr/RConn1 -- CF Track Terrain/RConn1 -- CF Track Bump 2/RConn1 -- CF Track Bump 4/RConn1 -- CF Track Bump 8/RConn1 -- CF Track Bump 6/RConn1

== system sm_excv_scene_lib/Flat Plane 1 Roller Spheres ==
  mL : Inport
  CF Roller Spheres Terrain L : sm_tracked_vehicle_lib/CF Roller Spheres Terrain Full  K_Road=Scene.Contact.Spheres.Terrain.K  B_Road=Scene.Contact.Spheres.Terrain.B  TW_Road=Scene.Contact.Spheres.Terrain.TW  F_dyn_Road=Scene.Contact.Spheres.Terrain.mud  F_stat_Road=Scene.Contact.Spheres.Terrain.mus  CV_Road=Scene.Contact.Spheres.Terrain.CV
  Infinite Plane : sm_lib/Curves and Surfaces/Infinite Plane  GraphicType=Rectangle  GraphicPlaneWidth=Scene.Plane.l  GraphicPlaneWidthUnits=m  GraphicPlaneHeight=Scene.Plane.w  GraphicPlaneHeightUnits=m  GraphicVisPropType=SimpleVisualProperties  GraphicDiffuseColor=[0.5 0.5 0.5]  GraphicOpacity=0.25  GraphicSpecularColor=[0.5 0.5 0.5 1.0]  GraphicAmbientColor=[0.15 0.15 0.15 1.0]  GraphicEmissiveColor=[0.0 0.0 0.0 1.0]  GraphicShininess=75
  Terminator : Terminator
  Transform Plane : sm_lib/Frames and Transforms/Rigid Transform  TranslationMethod=Cartesian  TranslationStandardOffset=0  TranslationStandardOffsetUnits=m  TranslationStandardAxis=+Z  TranslationCartesianOffset=Scene.Plane.offset  TranslationCartesianOffsetUnits=m  TranslationROffset=0  TranslationROffsetUnits=m  TranslationZOffset=0  TranslationZOffsetUnits=m  TranslationThetaOffset=0  TranslationThetaOffsetUnits=deg  RotationMethod=None  RotationAngleUnits=deg  RotationStandardAxis=+Z  RotationAngle=0.0  RotationArbitraryAxis=[0 0 1]  FollAlignAxisA=+X  BaseAlignAxisA=+Y  FollAlignAxisB=+Y  BaseAlignAxisB=+Z  RotationSequenceAxes=FollowerAxes  RotationSequence=XYX  RotationSequenceAngles=[0 0 0]  RotationSequenceAnglesUnits=deg  RotationMatrix=[1 0 0; 0 1 0; 0 0 1]  Quaternion=[1 0 0 0]
  L : PMIOPort  Side=Right
  W : PMIOPort  Port=2  Side=Right
  wires:
  mL/1 -> Terminator/1
  connections:
  Infinite Plane/RConn1 -- CF Roller Spheres Terrain L/LConn1
  L/RConn1 -- CF Roller Spheres Terrain L/RConn1
  Transform Plane/RConn1 -- Infinite Plane/LConn1
  Transform Plane/LConn1 -- W/RConn1

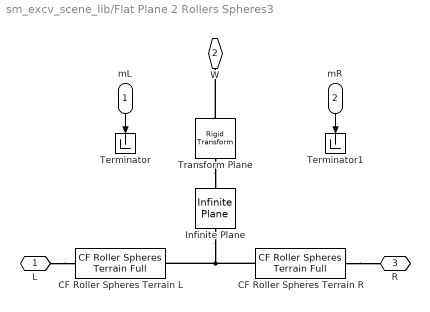
== system sm_excv_scene_lib/Flat Plane 2 Rollers Spheres3 ==
  mL : Inport
  mR : Inport  Port=2
  CF Roller Spheres Terrain L : sm_tracked_vehicle_lib/CF Roller Spheres Terrain Full  K_Road=Scene.Contact.Spheres.Terrain.K  B_Road=Scene.Contact.Spheres.Terrain.B  TW_Road=Scene.Contact.Spheres.Terrain.TW  F_dyn_Road=Scene.Contact.Spheres.Terrain.mud  F_stat_Road=Scene.Contact.Spheres.Terrain.mus  CV_Road=Scene.Contact.Spheres.Terrain.CV
  CF Roller Spheres Terrain R : sm_tracked_vehicle_lib/CF Roller Spheres Terrain Full  K_Road=Scene.Contact.Spheres.Terrain.K  B_Road=Scene.Contact.Spheres.Terrain.B  TW_Road=Scene.Contact.Spheres.Terrain.TW  F_dyn_Road=Scene.Contact.Spheres.Terrain.mud  F_stat_Road=Scene.Contact.Spheres.Terrain.mus  CV_Road=Scene.Contact.Spheres.Terrain.CV
  Infinite Plane : sm_lib/Curves and Surfaces/Infinite Plane  GraphicType=Rectangle  GraphicPlaneWidth=Scene.Plane.l  GraphicPlaneWidthUnits=m  GraphicPlaneHeight=Scene.Plane.w  GraphicPlaneHeightUnits=m  GraphicVisPropType=SimpleVisualProperties  GraphicDiffuseColor=[0.5 0.5 0.5]  GraphicOpacity=0.25  GraphicSpecularColor=[0.5 0.5 0.5 1.0]  GraphicAmbientColor=[0.15 0.15 0.15 1.0]  GraphicEmissiveColor=[0.0 0.0 0.0 1.0]  GraphicShininess=75
  Terminator : Terminator
  Terminator1 : Terminator
  Transform Plane : sm_lib/Frames and Transforms/Rigid Transform  TranslationMethod=Cartesian  TranslationStandardOffset=0  TranslationStandardOffsetUnits=m  TranslationStandardAxis=+Z  TranslationCartesianOffset=Scene.Plane.offset  TranslationCartesianOffsetUnits=m  TranslationROffset=0  TranslationROffsetUnits=m  TranslationZOffset=0  TranslationZOffsetUnits=m  TranslationThetaOffset=0  TranslationThetaOffsetUnits=deg  RotationMethod=None  RotationAngleUnits=deg  RotationStandardAxis=+Z  RotationAngle=0.0  RotationArbitraryAxis=[0 0 1]  FollAlignAxisA=+X  BaseAlignAxisA=+Y  FollAlignAxisB=+Y  BaseAlignAxisB=+Z  RotationSequenceAxes=FollowerAxes  RotationSequence=XYX  RotationSequenceAngles=[0 0 0]  RotationSequenceAnglesUnits=deg  RotationMatrix=[1 0 0; 0 1 0; 0 0 1]  Quaternion=[1 0 0 0]
  L : PMIOPort  Side=Right
  W : PMIOPort  Port=2  Side=Right
  R : PMIOPort  Port=3  Side=Right
  wires:
  mL/1 -> Terminator/1
  mR/1 -> Terminator1/1
  connections:
  Transform Plane/LConn1 -- W/RConn1
  Transform Plane/RConn1 -- Infinite Plane/LConn1
  L/RConn1 -- CF Roller Spheres Terrain L/RConn1
  CF Roller Spheres Terrain R/RConn1 -- R/RConn1
  CF Roller Spheres Terrain R/LConn1 -- Infinite Plane/RConn1 -- CF Roller Spheres Terrain L/LConn1

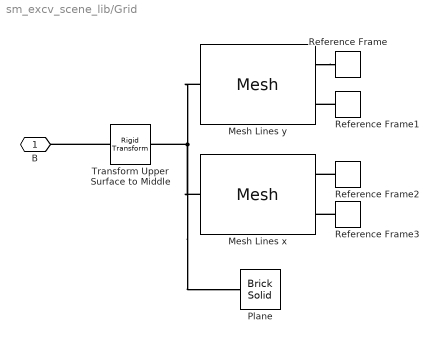
== system sm_excv_scene_lib/Grid ==
  Mesh Lines x : $bdroot/Mesh  mesh_lenx=grid_x  mesh_leny=grid_y  mesh_hx=hole_wy  mesh_hy=hole_ly  mesh_numhx=1  mesh_numhy=grid_num_sq_y  mesh_thickness=grid_z  mesh_rho=7000  mesh_color=grid_clr  mesh_opc=grid_opc
  "Mesh Lines y " : $bdroot/Mesh  mesh_lenx=grid_x  mesh_leny=grid_y  mesh_hx=hole_lx  mesh_hy=hole_wx  mesh_numhx=grid_num_sq_x  mesh_numhy=1  mesh_thickness=grid_z  mesh_rho=7000  mesh_color=grid_clr  mesh_opc=grid_opc
  Plane : sm_lib/Body Elements/Brick Solid  GraphicAmbientColor=[0.15 0.15 0.15 1.0]  BasedOnType=Density  BrickDimensions=[grid_x grid_y grid_z-0.01]  BrickDimensionsUnits=m  CenterOfMass=[0 0 0]  CenterOfMassUnits=m  GraphicDiffuseColor=[0.8 0.8 0.8]  Density=1000  DensityUnits=kg/m^3  DoExposeReferenceFrame=on  GraphicEmissiveColor=[0.0 0.0 0.0 1.0]  ExportEntireGeometry=off  SerializedFrames=<Frames/>  MarkerShape=Sphere  MarkerSize=10  GraphicType=FromGeometry  InertiaType=CalculateFromGeometry  Mass=1  MassUnits=kg  MomentsOfInertia=[1 1 1]  MomentsOfInertiaUnits=kg*m^2  GraphicOpacity=1.0  ProductsOfInertia=[0 0 0]  ProductsOfInertiaUnits=kg*m^2  GraphicShininess=75  GraphicSpecularColor=[0.5 0.5 0.5 1.0]  GraphicVisPropType=SimpleVisualProperties
  Reference Frame{,1..3} (4 alike) : sm_lib/Frames and Transforms/Reference Frame
  Transform Upper Surface to Middle : sm_lib/Frames and Transforms/Rigid Transform  TranslationMethod=StandardAxis  TranslationStandardOffset=-grid_z/2  TranslationStandardOffsetUnits=m  TranslationStandardAxis=+Z  TranslationCartesianOffset=[0 0 0]  TranslationCartesianOffsetUnits=m  TranslationROffset=0  TranslationROffsetUnits=m  TranslationZOffset=0  TranslationZOffsetUnits=m  TranslationThetaOffset=0  TranslationThetaOffsetUnits=deg  RotationMethod=None  RotationAngleUnits=deg  RotationStandardAxis=+Z  RotationAngle=0.0  RotationArbitraryAxis=[0 0 1]  FollAlignAxisA=+X  BaseAlignAxisA=+Y  FollAlignAxisB=+Y  BaseAlignAxisB=+Z  RotationSequenceAxes=FollowerAxes  RotationSequence=XYX  RotationSequenceAngles=[0 0 0]  RotationSequenceAnglesUnits=deg  RotationMatrix=[1 0 0; 0 1 0; 0 0 1]  Quaternion=[1 0 0 0]
  B : PMIOPort  Side=Right
  connections:
  Reference Frame3/RConn1 -- Mesh Lines x/RConn2
  "Mesh Lines y "/LConn1 -- Transform Upper Surface to Middle/RConn1 -- Mesh Lines x/LConn1 -- Plane/RConn1
  "Mesh Lines y "/RConn1 -- Reference Frame/RConn1
  Reference Frame1/RConn1 -- "Mesh Lines y "/RConn2
  Reference Frame2/RConn1 -- Mesh Lines x/RConn1
  Transform Upper Surface to Middle/LConn1 -- B/RConn1

== system sm_excv_scene_lib/Grid Surface Slope ==
  Grid Surface : sm_lib/Curves and Surfaces/Grid Surface  XGridVector=gs_data.xg  XGridVectorUnits=m  YGridVector=gs_data.yg  YGridVectorUnits=m  ZHeights=gs_data.zg  ZHeightsUnits=m  GraphicType=FromGeometry  GraphicVisPropType=SimpleVisualProperties  GraphicDiffuseColor=surface_clr  GraphicOpacity=surface_opc  GraphicSpecularColor=[0.5 0.5 0.5 1.0]  GraphicAmbientColor=[0.15 0.15 0.15 1.0]  GraphicEmissiveColor=[0.0 0.0 0.0 1.0]  GraphicShininess=75
  W : PMIOPort  Side=Right
  G : PMIOPort  Port=2  Side=Left
  connections:
  Grid Surface/RConn1 -- G/RConn1
  Grid Surface/LConn1 -- W/RConn1

== system sm_excv_scene_lib/Grid Surface Slope 1 Track ==
  CF Track Terrain L : sm_tracked_vehicle_lib/CF Track Terrain Full  K_Road=K_Road  B_Road=B_Road  TW_Road=TW_Road  F_dyn_Road=F_dyn_Road  F_stat_Road=F_stat_Road  CV_Road=CV_Road
      settings: LibrarySourceBlock=sm_chain_drive_lib/CF_Road_Full
  Grid Surface Slope : $bdroot/Grid Surface Slope  road_len=road_len  road_wid=road_wid  slope_run=slope_run  slope_rise=slope_rise  slope_x0=slope_x0  slope_xres=slope_xres  surface_clr=surface_clr  surface_opc=surface_opc
  W : PMIOPort  Side=Right
  L : PMIOPort  Port=2  Side=Left
  connections:
  CF Track Terrain L/RConn1 -- L/RConn1
  Grid Surface Slope/RConn1 -- W/RConn1
  Grid Surface Slope/LConn1 -- CF Track Terrain L/LConn1

== system sm_excv_scene_lib/Grid Surface Slope 2 Track ==
  CF Track Terrain L : sm_tracked_vehicle_lib/CF Track Terrain Full  K_Road=K_Road  B_Road=B_Road  TW_Road=TW_Road  F_dyn_Road=F_dyn_Road  F_stat_Road=F_stat_Road  CV_Road=CV_Road
      settings: LibrarySourceBlock=sm_chain_drive_lib/CF_Road_Full
  CF Track Terrain R : sm_tracked_vehicle_lib/CF Track Terrain Full  K_Road=K_Road  B_Road=B_Road  TW_Road=TW_Road  F_dyn_Road=F_dyn_Road  F_stat_Road=F_stat_Road  CV_Road=CV_Road
      settings: LibrarySourceBlock=sm_chain_drive_lib/CF_Road_Full
  Grid Surface Slope : $bdroot/Grid Surface Slope  road_len=road_len  road_wid=road_wid  slope_run=slope_run  slope_rise=slope_rise  slope_x0=slope_x0  slope_xres=slope_xres  surface_clr=surface_clr  surface_opc=surface_opc
  W : PMIOPort  Side=Right
  L : PMIOPort  Port=2  Side=Left
  R : PMIOPort  Port=3  Side=Left
  connections:
  CF Track Terrain R/LConn1 -- CF Track Terrain L/LConn1 -- Grid Surface Slope/LConn1
  R/RConn1 -- CF Track Terrain R/RConn1
  CF Track Terrain L/RConn1 -- L/RConn1
  Grid Surface Slope/RConn1 -- W/RConn1
